simulink model "three_ph_rect_buck"  (R2018a)
settings: Solver=VariableStepAuto  StartTime=-0.04  StopTime=0.02  MaxStep=4e-7  RelTol=1e-3
libraries: powerlib x20
settings Model: Creator=c  LastModifiedBy=pdb
settings DebuggingCC: UnconnectedOutputMsg=none

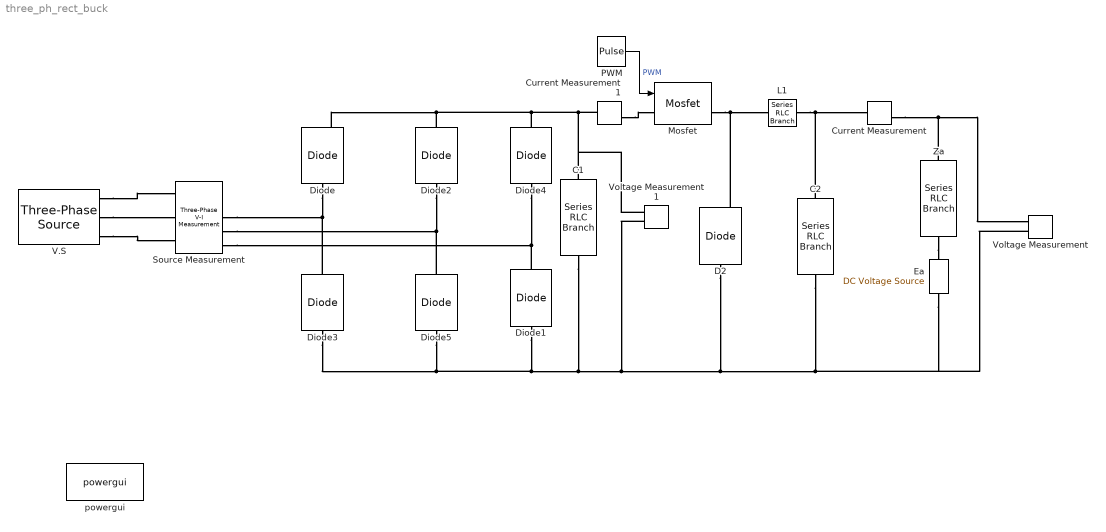
== system three_ph_rect_buck ==
  C1 : powerlib/Elements/Series RLC Branch  LConnTagsString=__new0  RConnTagsString=__new0  BranchType=C  Resistance=1  Inductance=1e-5  SetiL0=off  InitialCurrent=0  Capacitance=1e-3  Setx0=on  InitialVoltage=290  Measurements=None
  C2 : powerlib/Elements/Series RLC Branch  LConnTagsString=__new0  RConnTagsString=__new0  BranchType=C  Resistance=1  Inductance=1e-5  SetiL0=off  InitialCurrent=0  Capacitance=200e-6  Setx0=on  InitialVoltage=220  Measurements=None
  Current Measurement : powerlib/Measurements/Current Measurement  PhasorSimulation=off  OutputType=Complex  PSBequivalent=0
  Current Measurement1 : powerlib/Measurements/Current Measurement  PhasorSimulation=off  OutputType=Complex  PSBequivalent=0
  D2 : powerlib/Power Electronics/Diode  Ron=0.001  Lon=0  Vf=0.8  IC=0  UseSnubber=0  Rs=inf  Cs=0  Measurements=on
  Diode : powerlib/Power Electronics/Diode  Ron=0.001  Lon=0  Vf=0.8  IC=0  UseSnubber=0  Rs=inf  Cs=0  Measurements=on
  Diode{1..5} (5 alike) : powerlib/Power Electronics/Diode  Ron=0.001  Lon=0  Vf=0.8  IC=0  UseSnubber=0  Rs=inf  Cs=0  Measurements=off
  Ea : powerlib/Electrical Sources/DC Voltage Source  Amplitude=202  Measurements=None
  L1 : powerlib/Elements/Series RLC Branch  LConnTagsString=__new0  RConnTagsString=__new0  BranchType=L  Resistance=1e-3  Inductance=100e-6  SetiL0=off  InitialCurrent=0  Capacitance=1e-6  Setx0=off  InitialVoltage=0  Measurements=None
  Mosfet : powerlib/Power Electronics/Mosfet  Ron=0.1  Lon=0  Rd=0.01  Vfd=0  IC=0  Rs=10e3  Cs=0  Measurements=on
  PWM : DiscretePulseGenerator  PulseType=Time based  Period=1/10e3  PulseWidth=75  PhaseDelay=-10
  Source Measurement : powerlib/Measurements/Three-Phase V-I Measurement  VoltageMeasurement=phase-to-ground  SetLabelV=off  LabelV=Vabc  Vpu=off  VpuLL=off  CurrentMeasurement=yes  SetLabelI=off  LabelI=Iabc  Ipu=off  Pbase=100e6  Vbase=500e3  OutputType=Complex  PhasorSimulation=off  PSBequivalent=0
  V.S : powerlib/Electrical Sources/Three-Phase Source  InternalConnection=Yg  VoltagePhases=off  Voltage=120*sqrt(3)  PhaseAngle=0  Voltage_phases=[25e3 25e3 25e3]/sqrt(3)  PhaseAngles_phases=[0 -120 +120]  Frequency=50  NonIdealSource=on  SpecifyImpedance=off  Resistance=0.05  Inductance=1.8e-4  ShortCircuitLevel=sqrt(3)*220*20000  BaseVoltage=120*sqrt(3)  XRratio=0.1  BusType=swing  Pref=10e3  Qref=0  Prefabc=[10e3, 10e3, 10e3]  Qrefabc=[0, 0, 0]  Qmin=-inf  Qmax=inf
  Voltage Measurement : powerlib/Measurements/Voltage Measurement  PhasorSimulation=off  OutputType=Complex  PSBequivalent=0
  Voltage Measurement1 : powerlib/Measurements/Voltage Measurement  PhasorSimulation=off  OutputType=Complex  PSBequivalent=0
  Za : powerlib/Elements/Series RLC Branch  LConnTagsString=__new0  RConnTagsString=__new0  BranchType=RL  Resistance=0.8  Inductance=0.0125  SetiL0=on  InitialCurrent=16  Capacitance=1e-6  Setx0=off  InitialVoltage=0  Measurements=None
  powergui : powerlib/powergui  Priority=1  SimulationMode=Continuous  SampleTime=50e-6  frequency=60  Iterations=50  frequencyindice=0  Pbase=100e6  ErrMax=1e-4  UnitsV=kV  UnitsW=MW  buscounter=0  FunctionMessages=off  echomessages=off  EnableUseOfTLC=off  CurrentSourceSwitches=off  DisableSnubberDevices=off  DisableRonSwitches=off  DisableVfSwitches=off  DisplayEquations=off  SolverType=Tustin/Backward Euler (TBE)  Interpol=off  ExternalGateDelay=off  methode=off  Ts=100  x0status=blocks  SPID=on  SwTol=0  HookPort=off  RestoreLinks=warning  ResistiveCurrentMeasurement=off  Frange=[0:2:500]  Ylog=off  Xlog=on  ShowGrid=off  save=off  variable=ZData  structure=0  ZoomFFT=off  StartTime=0.0  cycles=1  DisplayStyle=1  fundamental=60  FreqAxis=off  MaxFrequency=1000  frequencyindicesteady=1  RmsSteady=1  display=off
  wires:
  PWM/1 -> Mosfet/1  "PWM"
  connections:
  Diode/RConn1 -- Current Measurement1/LConn1 -- Voltage Measurement1/LConn1 -- C1/LConn1 -- Diode4/RConn1 -- Diode2/RConn1
  Current Measurement/RConn1 -- Za/LConn1 -- Voltage Measurement/LConn1
  Source Measurement/RConn1 -- Diode3/RConn1 -- Diode/LConn1
  Source Measurement/RConn2 -- Diode5/RConn1 -- Diode2/LConn1
  V.S/RConn3 -- Source Measurement/LConn3
  V.S/RConn2 -- Source Measurement/LConn2
  V.S/RConn1 -- Source Measurement/LConn1
  Diode1/LConn1 -- Voltage Measurement1/LConn2 -- Ea/LConn1 -- Voltage Measurement/LConn2 -- C2/RConn1 -- D2/LConn1 -- C1/RConn1 -- Diode3/LConn1 -- Diode5/LConn1
  C2/LConn1 -- L1/RConn1 -- Current Measurement/LConn1
  Za/RConn1 -- Ea/RConn1
  D2/RConn1 -- Mosfet/RConn1 -- L1/LConn1
  Diode1/RConn1 -- Source Measurement/RConn3 -- Diode4/LConn1
  Current Measurement1/RConn1 -- Mosfet/LConn1
